simulink model "MOTOR_SHIELD_using_arduino_due"  (R2024b)
settings: Solver=FixedStepDiscrete  StartTime=0.0  StopTime=Inf  FixedStep=1/1000  RelTol=1e-3  EnableMultiTasking=on
libraries: dspstat3 x2, Du_Gimbal_LIB x1, arduinolib x1
settings Model: ExtModeTrigDuration=2  Creator=leoni  LastModifiedBy=leoni
settings SolverCC: AutoInsertRateTranBlk=on
settings OptimizationCC: EnhancedBackFolding=on  PassReuseOutputArgsAs=Individual arguments  ZeroExternalMemoryAtStartup=off  ZeroInternalMemoryAtStartup=off  MaxStackSize=64  OptimizeBlockOrder=speed  DifferentSizesBufferReuse=on  OptimizationCustomize=off  EfficientTunableParamExpr=on
settings DebuggingCC: ParameterTunabilityLossMsg=error
settings HardwareCC: ProdBitPerPointer=32  ProdBitPerSizeT=32  ProdBitPerPtrDiffT=32  ProdLargestAtomicInteger=Long  ProdLargestAtomicFloat=Double  ProdWordSize=32  ProdHWDeviceType=ARM Compatible->ARM Cortex
settings SFSimCC: MATLABDynamicMemAlloc=off
settings RTWCC: Description=Embedded Coder  SystemTargetFile=ert.tlc  HardwareBoard=Arduino Due  TemplateMakefile=ert_default_tmf  Toolchain=Arduino ARM  BuildConfiguration=Faster Runs
settings CodeAppCC: ForceParamTrailComments=on  IgnoreCustomStorageClasses=off  OperatorAnnotations=on  SimulinkDataObjDesc=on  SFDataObjDesc=on  InsertBlockDesc=on
settings ERTTargetCC: SupportContinuousTime=on  SupportVariableSizeSignals=on  ExtModeTransport=3  ExtModeStaticAlloc=on  ExtModeAutomaticAllocSize=off  ExtModeStaticAllocSize=24576  ExtModeMexFile=ext_xcp  ExtModeIntrfLevel=Level2 - Open  InlinedParameterPlacement=Hierarchical

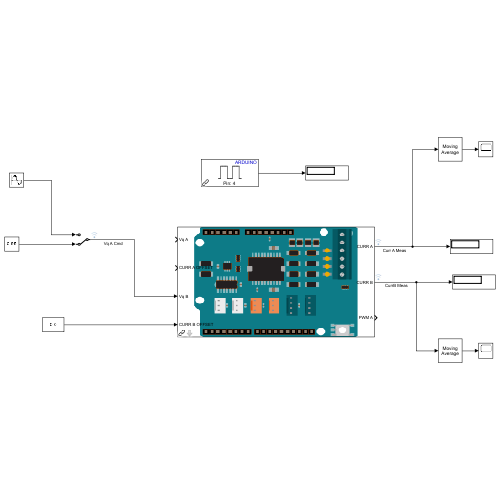
[thumbnail: Simulink's stored preview of the top-level diagram]
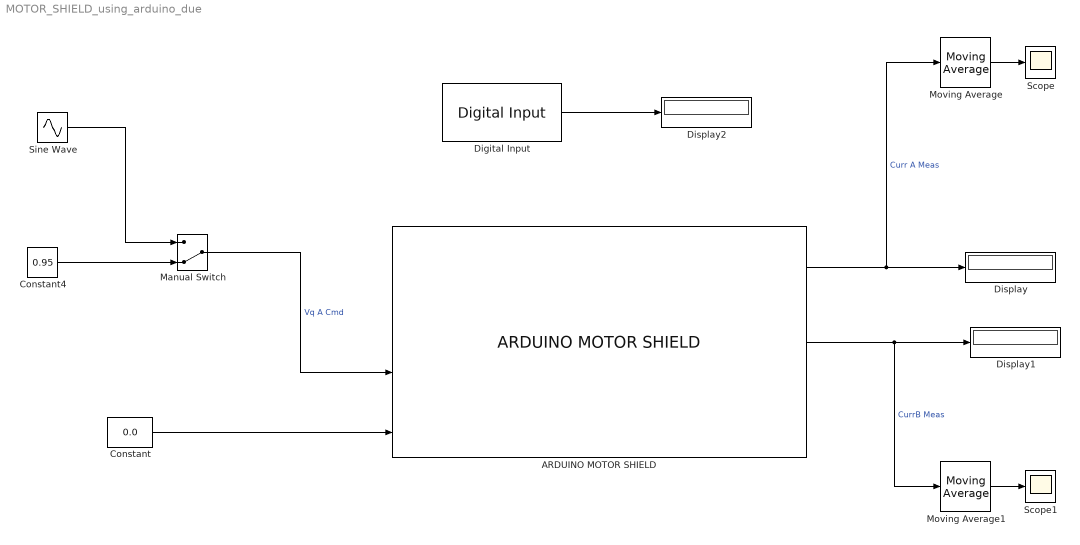
== system MOTOR_SHIELD_using_arduino_due ==
  ARDUINO MOTOR SHIELD : Du_Gimbal_LIB/ARDUINO MOTOR SHIELD  ts=0.01  VqMax=0.105  motAdirReverse=off  motBdirReverse=off
  Constant : Constant  Value=0.0
  Constant4 : Constant  Value=0.95  SampleTime=Inf
  Digital Input : arduinolib/Digital Input  pinNumber=4  mode=Default  Direction=input  SampleTime=0.1  blockPlatform=arduino
      settings: SourceProductName=Common
  Display : Display
  Display1 : Display
  Display2 : Display
  Manual Switch : ManualSwitch  CurrentSetting=0
  Moving Average : dspstat3/Moving Average  Method=Exponential weighting  ForgettingFactorPort=off  SpecifyWindowLength=on  WindowLength=4  OverlapLength=3  AllowArbitraryInputLength=off  ForgettingFactor=0.9  SimulateUsing=Interpreted execution
  Moving Average1 : dspstat3/Moving Average  Method=Exponential weighting  ForgettingFactorPort=off  SpecifyWindowLength=on  WindowLength=4  OverlapLength=3  AllowArbitraryInputLength=off  ForgettingFactor=0.9  SimulateUsing=Interpreted execution
  Scope : Scope
  Scope1 : Scope
  Sine Wave : Sin  Amplitude=10  Frequency=2*pi*1  SampleTime=0.005
  wires:
  Sine Wave/1 -> Manual Switch/1
  ARDUINO MOTOR SHIELD/1 -> Moving Average/1, Display/1  "Curr A Meas"
  Constant/1 -> ARDUINO MOTOR SHIELD/4
  Manual Switch/1 -> ARDUINO MOTOR SHIELD/3  "Vq A Cmd"
  Constant4/1 -> Manual Switch/2
  Moving Average/1 -> Scope/1
  ARDUINO MOTOR SHIELD/2 -> Moving Average1/1, Display1/1  "CurrB Meas"
  Moving Average1/1 -> Scope1/1
  Digital Input/1 -> Display2/1
